simulink model "inverse_kinematics_func_sim"  (R2023a)
settings: Solver=VariableStepAuto  StartTime=0.0  StopTime=10.0  RelTol=1e-3
settings Model: Creator=totae  LastModifiedBy=totae

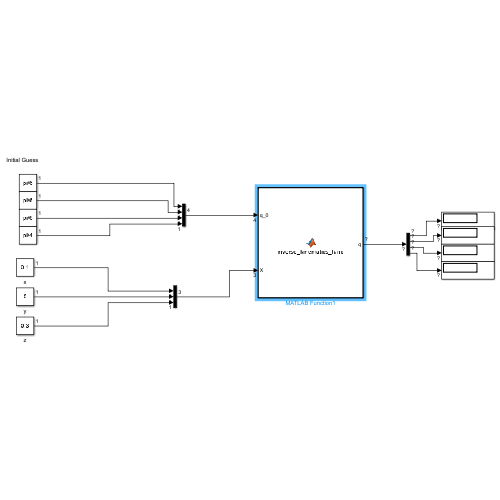
[thumbnail: Simulink's stored preview of the top-level diagram]
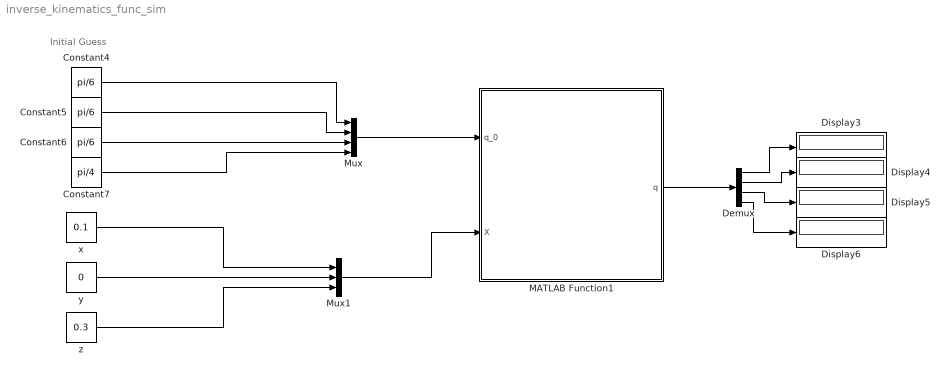
== system inverse_kinematics_func_sim ==
  note: Initial Guess
  Constant4 : Constant  Value=pi/6
  Constant5 : Constant  Value=pi/6
  Constant6 : Constant  Value=pi/6
  Constant7 : Constant  Value=pi/4
  Demux : Demux
  Display{3..6} (4 alike) : Display
  MATLAB Function1 : MATLAB Function  TreatAsAtomicUnit=on
  Mux : Mux
  Mux1 : Mux  Inputs=3
  x : Constant  Value=0.1
  y : Constant  Value=0
  z : Constant  Value=0.3
  wires:
  z/1 -> Mux1/3
  x/1 -> Mux1/1
  Constant4/1 -> Mux/1
  Constant5/1 -> Mux/2
  Mux/1 -> MATLAB Function1/1(q_0)
  y/1 -> Mux1/2
  Constant6/1 -> Mux/3
  Demux/1 -> Display3/1
  Constant7/1 -> Mux/4
  Demux/3 -> Display5/1
  Demux/4 -> Display6/1
  MATLAB Function1/1(q) -> Demux/1
  Demux/2 -> Display4/1
  Mux1/1 -> MATLAB Function1/2(X)

== matlab function inverse_kinematics_func_sim/MATLAB Function1 ==
  data: q_0 input; q output; X input
function q = inverse_kinematics_func(q_0, X)

q0 = coder.const('q0');
q1 = coder.const('q1');
q2 = coder.const('q2');
q3 = coder.const('q3');

[x,y,z]=forward_kinematics_func();
fq_n=[x-X(1),y-X(2),z-X(3)];
fq_n=subs(fq_n,q0,q_0(1));
fq_n=subs(fq_n,q1,q_0(2));
fq_n=subs(fq_n,q2,q_0(3));
fq_n=subs(fq_n,q3,q_0(4));
f_j = inverse_jacobian_matrix(q_0);
q_n=(q_0)-(f_j*transpose(fq_n));
i=0;
while(i<20)
q_0=q_n
fq_n=[x-X(1),y-X(2),z-X(3)];
fq_n=subs(fq_n,q0,q_0(1));
fq_n=subs(fq_n,q1,q_0(2));
fq_n=subs(fq_n,q2,q_0(3));
fq_n=subs(fq_n,q3,q_0(4));
f_j = inverse_jacobian_matrix(q_0);
q_n=q_0-(f_j*transpose(fq_n));
q_n=vpa(q_n,10);
i=i+1;
end    
q=vpa(q_n,4);
end
